simulink model "steeringSimulationSimplifiedWithFilter"  (R2015b)
settings: Solver=ode45  StartTime=0.0  StopTime=20  RelTol=1e-3
libraries: simulink x2
settings Model: Creator=vniel  LastModifiedBy=Thomas
settings DataIOCC: SaveFormat=Array
settings HardwareCC: ProdBitPerPointer=32  ProdLargestAtomicFloat=None  ProdIntDivRoundTo=Undefined  ProdEndianess=Unspecified  ProdWordSize=32  ProdHWDeviceType=32-bit Generic
settings GRTTargetCC: GeneratePreprocessorConditionals=Disable all
settings ConfigComp: CovModelRefEnable=Off

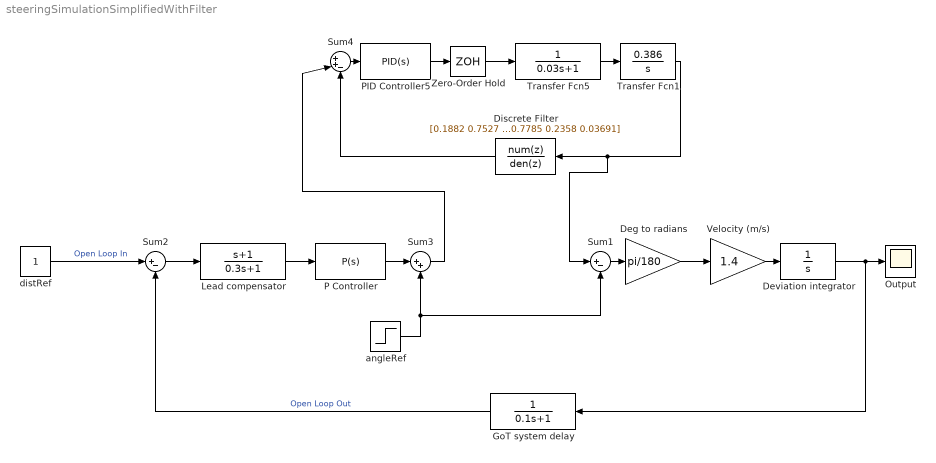
== system steeringSimulationSimplifiedWithFilter ==
  Deg to radians : Gain  Gain=pi/180
  Deviation integrator : TransferFcn  Denominator=[1 0]
  Discrete Filter : DiscreteFilter  Numerator=[0.1882 0.7527 1.129 0.7527 0.1882]  Denominator=[1 0.9595 0.7785 0.2358 0.03691]  SampleTime=0.015
  GoT system delay : TransferFcn  Denominator=[0.1 1]
  Lead compensator : TransferFcn  Numerator=[1 1]  Denominator=[0.3 1]
  Output : Scope
  P Controller : simulink/Continuous/PID Controller  Controller=P  TimeDomain=Continuous-time  SampleTime=-1  IntegratorMethod=Forward Euler  FilterMethod=Forward Euler  Form=Parallel  UseFilter=on  ControllerParametersSource=internal  P=48.87  I=0  D=0  N=0  InitialConditionSource=internal  InitialConditionForIntegrator=0  InitialConditionForFilter=0  ExternalReset=none  LimitOutput=on  UpperSaturationLimit=90  LowerSaturationLimit=-90  LinearizeAsGain=on  AntiWindupMode=none  Kb=1  TrackingMode=off  Kt=1  PParamMin=[]  PParamMax=[]  IParamMin=[]  IParamMax=[]  DParamMin=[]  DParamMax=[]  NParamMin=[]  NParamMax=[]  KbParamMin=[]  KbParamMax=[]  KtParamMin=[]  KtParamMax=[]  POutMin=[]  POutMax=[]  IOutMin=[]  IOutMax=[]  DOutMin=[]  DOutMax=[]  NOutMin=[]  NOutMax=[]  KbOutMin=[]  KbOutMax=[]  KtOutMin=[]  KtOutMax=[]  IntegratorOutMin=[]  IntegratorOutMax=[]  FilterOutMin=[]  FilterOutMax=[]  SumOutMin=[]  SumOutMax=[]  SumI1OutMin=[]  SumI1OutMax=[]  SumI2OutMin=[]  SumI2OutMax=[]  SumI3OutMin=[]  SumI3OutMax=[]  SumDOutMin=[]  SumDOutMax=[]  SaturationOutMin=[]  SaturationOutMax=[]  IntegratorContinuousStateAttributes=''  IntegratorStateMustResolveToSignalObject=off  IntegratorRTWStateStorageClass=Auto  FilterContinuousStateAttributes=''  FilterStateMustResolveToSignalObject=off  FilterRTWStateStorageClass=Auto  DifferentiatorICPrevScaledInput=0  DifferentiatorOutMin=[]  DifferentiatorOutMax=[]
  PID Controller5 : simulink/Continuous/PID Controller  Controller=PID  TimeDomain=Continuous-time  SampleTime=-1  IntegratorMethod=Forward Euler  FilterMethod=Forward Euler  Form=Parallel  UseFilter=on  ControllerParametersSource=internal  P=3  I=0  D=0  N=0  InitialConditionSource=internal  InitialConditionForIntegrator=0  InitialConditionForFilter=0  ExternalReset=none  LimitOutput=off  UpperSaturationLimit=7  LowerSaturationLimit=0  LinearizeAsGain=on  AntiWindupMode=none  Kb=1  TrackingMode=off  Kt=1  PParamMin=[]  PParamMax=[]  IParamMin=[]  IParamMax=[]  DParamMin=[]  DParamMax=[]  NParamMin=[]  NParamMax=[]  KbParamMin=[]  KbParamMax=[]  KtParamMin=[]  KtParamMax=[]  POutMin=[]  POutMax=[]  IOutMin=[]  IOutMax=[]  DOutMin=[]  DOutMax=[]  NOutMin=[]  NOutMax=[]  KbOutMin=[]  KbOutMax=[]  KtOutMin=[]  KtOutMax=[]  IntegratorOutMin=[]  IntegratorOutMax=[]  FilterOutMin=[]  FilterOutMax=[]  SumOutMin=[]  SumOutMax=[]  SumI1OutMin=[]  SumI1OutMax=[]  SumI2OutMin=[]  SumI2OutMax=[]  SumI3OutMin=[]  SumI3OutMax=[]  SumDOutMin=[]  SumDOutMax=[]  SaturationOutMin=[]  SaturationOutMax=[]  IntegratorContinuousStateAttributes=''  IntegratorStateMustResolveToSignalObject=off  IntegratorRTWStateStorageClass=Auto  FilterContinuousStateAttributes=''  FilterStateMustResolveToSignalObject=off  FilterRTWStateStorageClass=Auto  DifferentiatorICPrevScaledInput=0  DifferentiatorOutMin=[]  DifferentiatorOutMax=[]
  Sum1 : Sum  Inputs=|+-
  Sum2 : Sum  Inputs=|+-
  Sum3 : Sum  Inputs=|++
  Sum4 : Sum  Inputs=|++-
  Transfer Fcn1 : TransferFcn  Numerator=[0.386]  Denominator=[1 0]
  Transfer Fcn5 : TransferFcn  Denominator=[0.03 1]
  Velocity (m/s) : Gain  Gain=1.4
  Zero-Order Hold : ZeroOrderHold  SampleTime=0.015
  angleRef : Step  Time=5  After=0  SampleTime=0
  distRef : Constant
  wires:
  angleRef/1 -> Sum1/2, Sum3/2
  distRef/1 -> Sum2/1  "Open Loop In"
  Velocity (m/s)/1 -> Deviation integrator/1
  Sum1/1 -> Deg to radians/1
  P Controller/1 -> Sum3/1
  Deviation integrator/1 -> GoT system delay/1, Output/1
  GoT system delay/1 -> Sum2/2  "Open Loop Out"
  Transfer Fcn1/1 -> Sum1/1, Discrete Filter/1
  Sum2/1 -> Lead compensator/1
  Deg to radians/1 -> Velocity (m/s)/1
  Lead compensator/1 -> P Controller/1
  Transfer Fcn5/1 -> Transfer Fcn1/1
  Sum4/1 -> PID Controller5/1
  PID Controller5/1 -> Zero-Order Hold/1
  Discrete Filter/1 -> Sum4/3
  Sum3/1 -> Sum4/2
  Zero-Order Hold/1 -> Transfer Fcn5/1
